simulink model "Kalman_filter"  (R2024a)
settings: Solver=VariableStepAuto  StartTime=0.0  StopTime=0.3  RelTol=1e-3

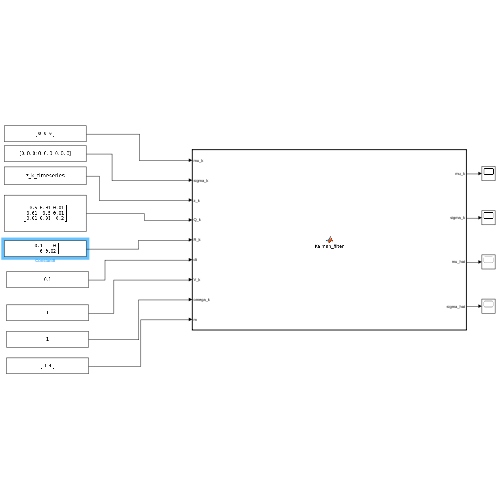
[thumbnail: Simulink's stored preview of the top-level diagram]
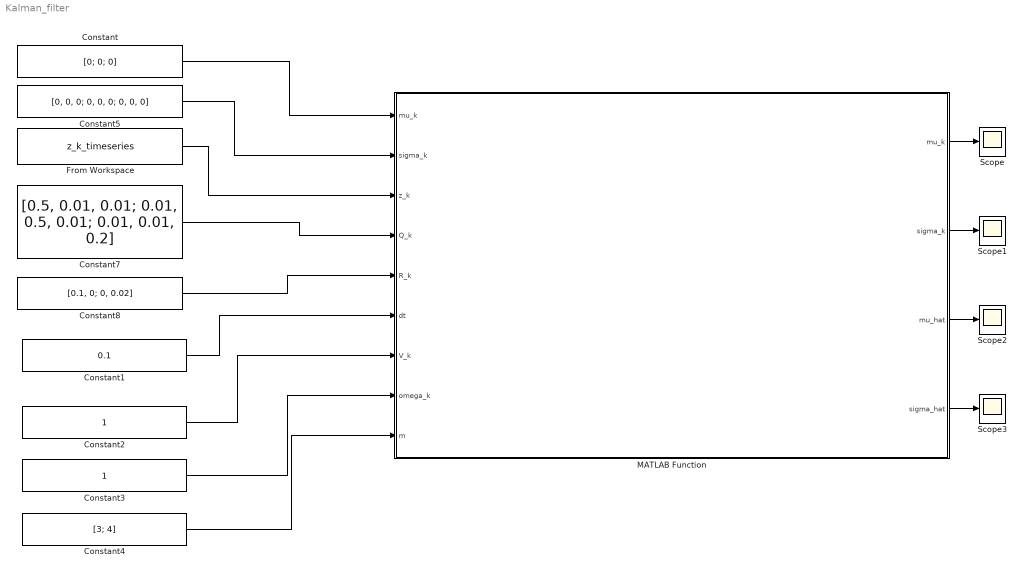
== system Kalman_filter ==
  Constant : Constant  Value=[0; 0; 0]
  Constant1 : Constant  Value=0.1
  Constant2 : Constant
  Constant3 : Constant
  Constant4 : Constant  Value=[3; 4]
  Constant5 : Constant  Value=[0, 0, 0; 0, 0, 0; 0, 0, 0]
  Constant7 : Constant  Value=[0.5, 0.01, 0.01; 0.01, 0.5, 0.01; 0.01, 0.01, 0.2]
  Constant8 : Constant  Value=[0.1, 0; 0, 0.02]
  From Workspace : FromWorkspace  VariableName=z_k_timeseries  SampleTime=0.1
  MATLAB Function : MATLAB Function  TreatAsAtomicUnit=on
  Scope{,1..3} (4 alike) : Scope
  wires:
  Constant4/1 -> MATLAB Function/9(m)
  Constant3/1 -> MATLAB Function/8(omega_k)
  Constant2/1 -> MATLAB Function/7(V_k)
  Constant1/1 -> MATLAB Function/6(dt)
  Constant/1 -> MATLAB Function/1("mu_k ")
  Constant5/1 -> MATLAB Function/2("sigma_k ")
  Constant7/1 -> MATLAB Function/4(Q_k)
  Constant8/1 -> MATLAB Function/5(R_k)
  MATLAB Function/1(mu_k) -> Scope/1
  MATLAB Function/4(sigma_hat) -> Scope3/1
  MATLAB Function/3(mu_hat) -> Scope2/1
  MATLAB Function/2(sigma_k) -> Scope1/1
  From Workspace/1 -> MATLAB Function/3(z_k)

== matlab function Kalman_filter/MATLAB Function ==
  data: mu_k input; mu_k output; sigma_k input; z_k input; Q_k input; R_k input; dt input; V_k input; omega_k input; m input; sigma_k output; mu_hat output; sigma_hat output
function [mu_k, sigma_k, mu_hat, sigma_hat] = Kalman_filter(mu_k, sigma_k, z_k, Q_k, R_k, dt, V_k, omega_k, m)
%#codegen

    % Predicción -- Dead Reckoning
    % PASO 2 - Calcular la posición estimada del robot
    step = [dt*V_k*cos(mu_k(3));
            dt*V_k*sin(mu_k(3));
            dt*omega_k];
    mu_hat = mu_k + step;

    % PASO 3 - Calcular el modelo linealizado usando propagación de incertidumbre (Jacobiano)
    H = [1, 0, -dt*V_k*sin(mu_k(3));
         0, 1, dt*V_k*cos(mu_k(3));
         0, 0, 1];

    % PASO 4 - Calcular propagación de la incertidumbre
    sigma_hat = H * sigma_k * H' + Q_k;

    % Corrección / Modelo de observación

    % PASO 5 - Calcular error al landmark (Medida real)
    delta = m - mu_hat(1:2);

    % PASO 6 - Calcular medida con el Modelo de observación
    z_hat = [sqrt(sum(delta.^2));
             atan2(delta(2), delta(1)) - mu_hat(3)];

    % PASO 7 - Linealizar el Modelo de observación
    G = [-delta(1)/(sqrt(sum(delta.^2))), -delta(2)/(sqrt(sum(delta.^2))), 0;
         delta(2)/(sum(delta.^2)), -delta(1)/(sum(delta.^2)), -1];

    % PASO 8 - Incertidumbre de la medición
    Z = G * sigma_hat * G' + R_k;

    % PASO 9 - Ganancia de kalman 
    K = sigma_hat * G' / Z;

    % PASO 10 - Calcular la posición del robot usando la observación real z_i
    mu_k = mu_hat + K * (z_k - z_hat);

    % PASO 10 - Calcular covarianza
    sigma_k = (eye(3) - K * G) * sigma_hat;
end

%{
%Mediciones lidar declaradas en workspace para cada iteracion
% Definir las mediciones y los tiempos de muestreo
z_k_list = { [4.87; 0.8], [4.72; 0.72], [4.69; 0.65] };
time = [0.1, 0.2, 0.3]; % tiempos de muestreo correspondientes

% Convertir las mediciones a una matriz
data = [z_k_list{:}]'; % Transponer para obtener una matriz de 3x2

% Crear el objeto timeseries
z_k_timeseries = timeseries(data, time);

% Mostrar para verificación
disp(z_k_timeseries);
%}
